simulink model "Testbench_Arch"  (R2022b)
settings: Solver=FixedStepDiscrete  StartTime=0.0  StopTime=10.0  RelTol=1e-3
undefined symbols (not defined in the file or in its folder): D1, P
settings Model: Creator=MAAM  LastModifiedBy=MAAM

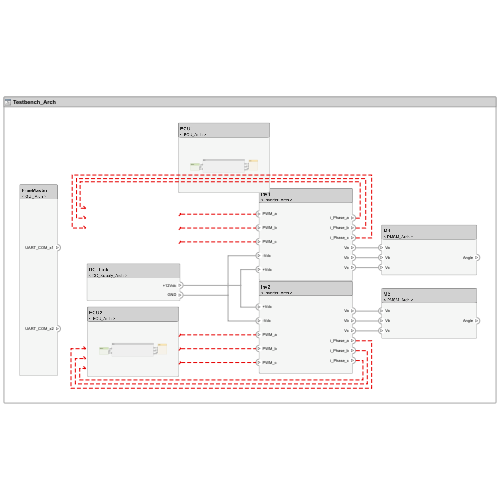
[thumbnail: Simulink's stored preview of the top-level diagram]
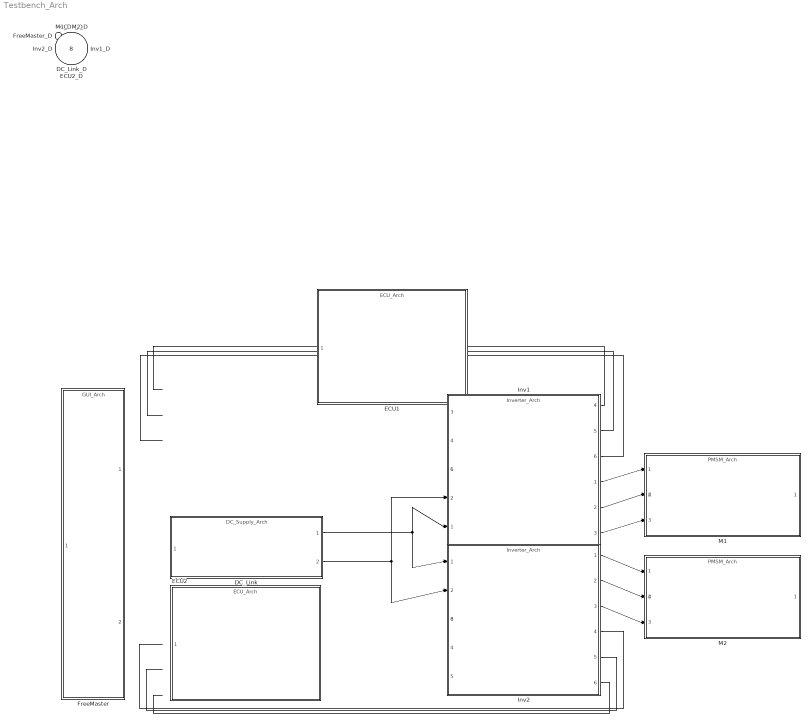
== system Testbench_Arch ==
  DC_Link_D : Inport  OutputFunctionCall=on
  ECU1_D : Inport  Port=2  OutputFunctionCall=on
  ECU2_D : Inport  Port=3  OutputFunctionCall=on
  FreeMaster_D : Inport  Port=4  OutputFunctionCall=on
  Inv1_D : Inport  Port=5  OutputFunctionCall=on
  Inv2_D : Inport  Port=6  OutputFunctionCall=on
  M1_D : Inport  Port=7  OutputFunctionCall=on
  M2_D : Inport  Port=8  OutputFunctionCall=on
  DC_Link : ModelReference  ModelNameDialog=DC_Supply_Arch.slx  SimulationMode=Normal  ScheduleRates=on  ModelEventPortInfo=P:D1[-2][0][0]  ModelReferenceVersion=1.3
      settings: PortSchema="{\"entries\":[{\"content\":{\"headerSize\":38,\"margin\":15,\"minimumSpacing\":25,\"sides\":[{\"content\":{\"connectorIds\":[]},\"type\":\"ConnectorPlacement.EquallySpacedRectSide\",\"uuid\":\"fed1c8e5-ca43-4606-b1ad-f0c744bc55d4\"},{\"content\":{\"connectorIds\":[\"Out1\",\"Out2\"],\"side\":\"RIGHT\"},\"type\":\"ConnectorPlacement.EquallySpacedRectSide\",\"uuid\":\"4b4c2077-2e65-4c1c-92f5-83c29014d170\"},{\"content\":{\"connectorIds\":[],\"side\":\"TOP\"},\"type\":\"ConnectorPlacement.EquallySpacedRectSide\",\"uuid\":\"cd558f9c-4ef0-426f-b395-6a6bbc45ebcf\"},{\"content\":{\"connectorIds\":[\"In1\"],\"side\":\"HIDDEN\"},\"type\":\"ConnectorPlacement.EquallySpacedRectSide\",\"uuid\":\"73d34b5e-c1c3-4db8-959f-9188fb95aa52\"}]},\"type\":\"ConnectorPlacement.EquallySpacedConnector\",\"uuid\":\"0512200b-6013-4a9c-b2f2-e98bdb0370d1\"}],\"packageUris\":[\"http://schema.mathworks.com/mf0/Connector/R2020b\"],\"version\":\"1.0\"}"
  ECU1 : ModelReference  ModelNameDialog=ECU_Arch.slx  SimulationMode=Normal  ScheduleRates=on  ModelEventPortInfo=P:D1[-2][0][0]  ModelReferenceVersion=1.40
      settings: PortSchema="{\"entries\":[{\"content\":{\"headerSize\":38,\"margin\":15,\"minimumSpacing\":25,\"sides\":[{\"content\":{\"connectorIds\":[]},\"type\":\"ConnectorPlacement.EquallySpacedRectSide\",\"uuid\":\"fed1c8e5-ca43-4606-b1ad-f0c744bc55d4\"},{\"content\":{\"connectorIds\":[],\"side\":\"RIGHT\"},\"type\":\"ConnectorPlacement.EquallySpacedRectSide\",\"uuid\":\"4b4c2077-2e65-4c1c-92f5-83c29014d170\"},{\"content\":{\"connectorIds\":[],\"side\":\"TOP\"},\"type\":\"ConnectorPlacement.EquallySpacedRectSide\",\"uuid\":\"cd558f9c-4ef0-426f-b395-6a6bbc45ebcf\"},{\"content\":{\"connectorIds\":[\"In1\"],\"side\":\"HIDDEN\"},\"type\":\"ConnectorPlacement.EquallySpacedRectSide\",\"uuid\":\"d4d03c1e-8576-4030-a054-73c8d58f0937\"}]},\"type\":\"ConnectorPlacement.EquallySpacedConnector\",\"uuid\":\"0512200b-6013-4a9c-b2f2-e98bdb0370d1\"}],\"packageUris\":[\"http://schema.mathworks.com/mf0/Connector/R2020b\"],\"version\":\"1.0\"}"
  ECU2 : ModelReference  ModelNameDialog=ECU_Arch.slx  SimulationMode=Normal  ScheduleRates=on  ModelEventPortInfo=P:D1[-2][0][0]  ModelReferenceVersion=1.40
      settings: PortSchema="{\"entries\":[{\"content\":{\"headerSize\":38,\"margin\":15,\"minimumSpacing\":25,\"sides\":[{\"content\":{\"connectorIds\":[]},\"type\":\"ConnectorPlacement.EquallySpacedRectSide\",\"uuid\":\"fed1c8e5-ca43-4606-b1ad-f0c744bc55d4\"},{\"content\":{\"connectorIds\":[],\"side\":\"RIGHT\"},\"type\":\"ConnectorPlacement.EquallySpacedRectSide\",\"uuid\":\"4b4c2077-2e65-4c1c-92f5-83c29014d170\"},{\"content\":{\"connectorIds\":[],\"side\":\"TOP\"},\"type\":\"ConnectorPlacement.EquallySpacedRectSide\",\"uuid\":\"cd558f9c-4ef0-426f-b395-6a6bbc45ebcf\"},{\"content\":{\"connectorIds\":[\"In1\"],\"side\":\"HIDDEN\"},\"type\":\"ConnectorPlacement.EquallySpacedRectSide\",\"uuid\":\"d4d03c1e-8576-4030-a054-73c8d58f0937\"}]},\"type\":\"ConnectorPlacement.EquallySpacedConnector\",\"uuid\":\"0512200b-6013-4a9c-b2f2-e98bdb0370d1\"}],\"packageUris\":[\"http://schema.mathworks.com/mf0/Connector/R2020b\"],\"version\":\"1.0\"}"
  FreeMaster : ModelReference  ModelNameDialog=GUI_Arch.slx  SimulationMode=Normal  ScheduleRates=on  ModelEventPortInfo=P:D1[-2][0][0]  ModelReferenceVersion=1.2
      settings: PortSchema="{\"entries\":[{\"content\":{\"headerSize\":38,\"margin\":15,\"minimumSpacing\":25,\"sides\":[{\"content\":{\"connectorIds\":[]},\"type\":\"ConnectorPlacement.EquallySpacedRectSide\",\"uuid\":\"fed1c8e5-ca43-4606-b1ad-f0c744bc55d4\"},{\"content\":{\"connectorIds\":[\"Out1\",\"Out2\"],\"side\":\"RIGHT\"},\"type\":\"ConnectorPlacement.EquallySpacedRectSide\",\"uuid\":\"4b4c2077-2e65-4c1c-92f5-83c29014d170\"},{\"content\":{\"connectorIds\":[],\"side\":\"TOP\"},\"type\":\"ConnectorPlacement.EquallySpacedRectSide\",\"uuid\":\"cd558f9c-4ef0-426f-b395-6a6bbc45ebcf\"},{\"content\":{\"connectorIds\":[\"In1\"],\"side\":\"HIDDEN\"},\"type\":\"ConnectorPlacement.EquallySpacedRectSide\",\"uuid\":\"73d34b5e-c1c3-4db8-959f-9188fb95aa52\"}]},\"type\":\"ConnectorPlacement.EquallySpacedConnector\",\"uuid\":\"0512200b-6013-4a9c-b2f2-e98bdb0370d1\"}],\"packageUris\":[\"http://schema.mathworks.com/mf0/Connector/R2020b\"],\"version\":\"1.0\"}"
  Inv1 : ModelReference  ModelNameDialog=Inverter_Arch  SimulationMode=Normal  ScheduleRates=on  ModelEventPortInfo=P:D1[-2][0][0]  ModelReferenceVersion=1.4
      settings: PortSchema="{\"entries\":[{\"content\":{\"headerSize\":38,\"margin\":15,\"minimumSpacing\":25,\"sides\":[{\"content\":{\"connectorIds\":[\"In3\",\"In4\",\"In5\",\"In2\",\"In1\"]},\"type\":\"ConnectorPlacement.EquallySpacedRectSide\",\"uuid\":\"fed1c8e5-ca43-4606-b1ad-f0c744bc55d4\"},{\"content\":{\"connectorIds\":[\"Out4\",\"Out5\",\"Out6\",\"Out1\",\"Out2\",\"Out3\"],\"side\":\"RIGHT\"},\"type\":\"ConnectorPlacement.EquallySpacedRectSide\",\"uuid\":\"4b4c2077-2e65-4c1c-92f5-83c29014d170\"},{\"content\":{\"connectorIds\":[],\"side\":\"TOP\"},\"type\":\"ConnectorPlacement.EquallySpacedRectSide\",\"uuid\":\"cd558f9c-4ef0-426f-b395-6a6bbc45ebcf\"},{\"content\":{\"connectorIds\":[\"In6\"],\"side\":\"HIDDEN\"},\"type\":\"ConnectorPlacement.EquallySpacedRectSide\",\"uuid\":\"c2dc8d66-d9ee-421e-a7fc-2327caa6cbe4\"}]},\"type\":\"ConnectorPlacement.EquallySpacedConnector\",\"uuid\":\"0512200b-6013-4a9c-b2f2-e98bdb0370d1\"}],\"packageUris\":[\"http://schema.mathworks.com/mf0/Connector/R2020b\"],\"version\":\"1.0\"}"
  Inv2 : ModelReference  ModelNameDialog=Inverter_Arch  SimulationMode=Normal  ScheduleRates=on  ModelEventPortInfo=P:D1[-2][0][0]  ModelReferenceVersion=1.4
      settings: PortSchema="{\"entries\":[{\"content\":{\"headerSize\":38,\"margin\":15,\"minimumSpacing\":25,\"sides\":[{\"content\":{\"connectorIds\":[\"In1\",\"In2\",\"In3\",\"In4\",\"In5\"]},\"type\":\"ConnectorPlacement.EquallySpacedRectSide\",\"uuid\":\"fed1c8e5-ca43-4606-b1ad-f0c744bc55d4\"},{\"content\":{\"connectorIds\":[\"Out1\",\"Out2\",\"Out3\",\"Out4\",\"Out5\",\"Out6\"],\"side\":\"RIGHT\"},\"type\":\"ConnectorPlacement.EquallySpacedRectSide\",\"uuid\":\"4b4c2077-2e65-4c1c-92f5-83c29014d170\"},{\"content\":{\"connectorIds\":[],\"side\":\"TOP\"},\"type\":\"ConnectorPlacement.EquallySpacedRectSide\",\"uuid\":\"cd558f9c-4ef0-426f-b395-6a6bbc45ebcf\"},{\"content\":{\"connectorIds\":[\"In6\"],\"side\":\"HIDDEN\"},\"type\":\"ConnectorPlacement.EquallySpacedRectSide\",\"uuid\":\"c2dc8d66-d9ee-421e-a7fc-2327caa6cbe4\"}]},\"type\":\"ConnectorPlacement.EquallySpacedConnector\",\"uuid\":\"0512200b-6013-4a9c-b2f2-e98bdb0370d1\"}],\"packageUris\":[\"http://schema.mathworks.com/mf0/Connector/R2020b\"],\"version\":\"1.0\"}"
  M1 : ModelReference  ModelNameDialog=PMSM_Arch.slx  SimulationMode=Normal  ScheduleRates=on  ModelEventPortInfo=P:D1[-2][0][0]  ModelReferenceVersion=1.1
      settings: PortSchema="{\"entries\":[{\"content\":{\"headerSize\":38,\"margin\":15,\"minimumSpacing\":25,\"sides\":[{\"content\":{\"connectorIds\":[\"In1\",\"In2\",\"In3\"]},\"type\":\"ConnectorPlacement.EquallySpacedRectSide\",\"uuid\":\"fed1c8e5-ca43-4606-b1ad-f0c744bc55d4\"},{\"content\":{\"connectorIds\":[\"Out1\"],\"side\":\"RIGHT\"},\"type\":\"ConnectorPlacement.EquallySpacedRectSide\",\"uuid\":\"4b4c2077-2e65-4c1c-92f5-83c29014d170\"},{\"content\":{\"connectorIds\":[],\"side\":\"TOP\"},\"type\":\"ConnectorPlacement.EquallySpacedRectSide\",\"uuid\":\"cd558f9c-4ef0-426f-b395-6a6bbc45ebcf\"},{\"content\":{\"connectorIds\":[\"In4\"],\"side\":\"HIDDEN\"},\"type\":\"ConnectorPlacement.EquallySpacedRectSide\",\"uuid\":\"0fbce530-9109-4027-a322-78a8e6c22d86\"}]},\"type\":\"ConnectorPlacement.EquallySpacedConnector\",\"uuid\":\"0512200b-6013-4a9c-b2f2-e98bdb0370d1\"}],\"packageUris\":[\"http://schema.mathworks.com/mf0/Connector/R2020b\"],\"version\":\"1.0\"}"
  M2 : ModelReference  ModelNameDialog=PMSM_Arch  SimulationMode=Normal  ScheduleRates=on  ModelEventPortInfo=P:D1[-2][0][0]  ModelReferenceVersion=1.1
      settings: PortSchema="{\"entries\":[{\"content\":{\"headerSize\":38,\"margin\":15,\"minimumSpacing\":25,\"sides\":[{\"content\":{\"connectorIds\":[\"In1\",\"In2\",\"In3\"]},\"type\":\"ConnectorPlacement.EquallySpacedRectSide\",\"uuid\":\"fed1c8e5-ca43-4606-b1ad-f0c744bc55d4\"},{\"content\":{\"connectorIds\":[\"Out1\"],\"side\":\"RIGHT\"},\"type\":\"ConnectorPlacement.EquallySpacedRectSide\",\"uuid\":\"4b4c2077-2e65-4c1c-92f5-83c29014d170\"},{\"content\":{\"connectorIds\":[],\"side\":\"TOP\"},\"type\":\"ConnectorPlacement.EquallySpacedRectSide\",\"uuid\":\"cd558f9c-4ef0-426f-b395-6a6bbc45ebcf\"},{\"content\":{\"connectorIds\":[\"In4\"],\"side\":\"HIDDEN\"},\"type\":\"ConnectorPlacement.EquallySpacedRectSide\",\"uuid\":\"0fbce530-9109-4027-a322-78a8e6c22d86\"}]},\"type\":\"ConnectorPlacement.EquallySpacedConnector\",\"uuid\":\"0512200b-6013-4a9c-b2f2-e98bdb0370d1\"}],\"packageUris\":[\"http://schema.mathworks.com/mf0/Connector/R2020b\"],\"version\":\"1.0\"}"
  wires:
  DC_Link/2 -> Inv2/2, Inv1/2
  DC_Link/1 -> Inv2/1, Inv1/1
  Inv1/3 -> M1/3
  Inv1/2 -> M1/2
  Inv1/1 -> M1/1
  Inv2/4 -> ?
  Inv2/5 -> ?
  Inv2/1 -> M2/1
  Inv2/6 -> ?
  ? -> Inv2/5
  Inv2/3 -> M2/3
  Inv2/2 -> M2/2
  ? -> Inv2/3
  ? -> Inv2/4
  ? -> Inv1/3
  ? -> Inv1/4
  ? -> Inv1/5
  Inv1/6 -> ?
  Inv1/5 -> ?
  Inv1/4 -> ?
